simulink model "FFT_FILTER_DESIGN"  (R2020b)
settings: Solver=VariableStepAuto  StartTime=0.0  StopTime=inf  RelTol=1e-3
libraries: dspsrcs4 x2, dspxfrm3 x2, commrandsrc3 x1, simulink x1, commutil2 x1, dspmathops x1
settings Model: Creator=Qrush  LastModifiedBy=AlexKurash

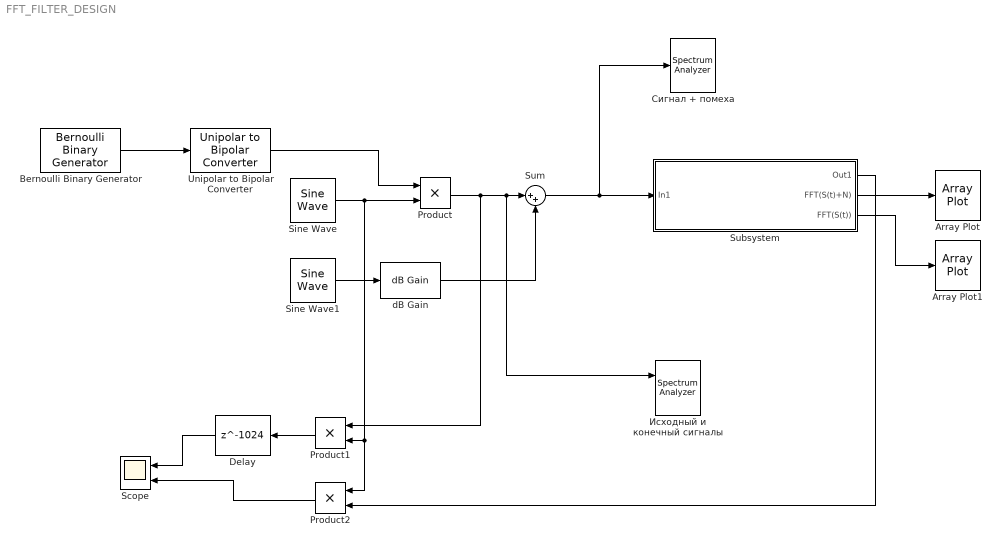
== system FFT_FILTER_DESIGN ==
  Array Plot : ArrayPlot
  Array Plot1 : ArrayPlot
  Bernoulli Binary Generator : commrandsrc3/Bernoulli Binary Generator  ProbabilityOfZero=0.5  SeedSource=Auto  Seed=0  SampleTime=1/128  SamplesPerFrame=1  OutputDataType=double  SimulateUsing=Interpreted execution
  Delay : Delay  DelayLength=1024  InitialCondition=0
  Product : Product
  Product1 : Product
  Product2 : Product
  Scope : Scope  NumInputPorts=2
  Sine Wave : dspsrcs4/Sine Wave  Amplitude=1  Frequency=200  Phase=0  SampleMode=Discrete  OutComplex=Real  CompMethod=Trigonometric fcn  TableSize=Speed  SampleTime=1/2048  SamplesPerFrame=1  ResetState=Restart at time zero  OutputFrames=off  dataType=double  wordLen=16  udDataType=sfix(16)  fracBitsMode=Best precision  numFracBits=15  OutDataTypeStr=double  LastOutDataTypeStr=double
  Sine Wave1 : dspsrcs4/Sine Wave  Amplitude=1  Frequency=224  Phase=0  SampleMode=Discrete  OutComplex=Real  CompMethod=Trigonometric fcn  TableSize=Speed  SampleTime=1/2048  SamplesPerFrame=1  ResetState=Restart at time zero  OutputFrames=off  dataType=double  wordLen=16  udDataType=sfix(16)  fracBitsMode=Best precision  numFracBits=15  OutDataTypeStr=double  LastOutDataTypeStr=double
  Subsystem : Subsystem  mask(Fourier Filtration){FFT_Length=1024, ThrValue=150}
      mask prompts: FFT_Length "FFT Length (число точек БПФ):"; ThrValue "Thresshold Value (Пороговое Значение)"
      mask help:
      | ENG: This block performs bandpass interference rejection based on the fast Fourier transform algorithm, the rejection is performed by comparing the components with the threshold level, and zeroing the components that exceed the specified threshold.
      |
      | The threshold level can be set based on graphically visualized FFT results that can be obtained from the debug ports.
      | ----------------------------------------
      | RUS: Данный блок осуществляет режекцию полосовых помех на основании алгоритма быстрого преобразования фурье, режекция осуществляется путем сравнения компонент с пороговым уровнем, и обнулением компоненты превышающих заданный порог.
      |
      | Настройку порогового уровня можно осуществить на основании графически-визуализированных результатов FFT , которые могут быть получены с портов отладки
      | ----------------------------------------
      mask Display:
      | disp ('FFT filtration')
      | port_label('input', 1, 'S(t)+N')
      | port_label('output', 1, 'S(t)')
      | port_label('output', 2, 'FFT(S(t)+N)')
      | port_label('output', 3, 'FFT(S(t))')
  Sum : Sum  Inputs=|++
  Unipolar to Bipolar Converter : commutil2/Unipolar to Bipolar Converter  M=2  polarity=Positive  dataType=Inherit via internal rule
  dB Gain : dspmathops/dB Gain  dB=-5  intype=Power
      settings: SourceProductBaseCode=DS
  Исходный и конечный сигналы : SpectrumAnalyzer  NumInputPorts=2
  Сигнал + помеха : SpectrumAnalyzer
  wires:
  Sine Wave1/1 -> dB Gain/1
  Sine Wave/1 -> Product2/1, Product1/2, Product/2
  Product/1 -> Product1/1, Исходный и конечный сигналы/1, Sum/1
  Bernoulli Binary Generator/1 -> Unipolar to Bipolar Converter/1
  Unipolar to Bipolar Converter/1 -> Product/1
  Sum/1 -> Subsystem/1(In1), Сигнал + помеха/1
  Product1/1 -> Delay/1
  Delay/1 -> Scope/1
  Product2/1 -> Scope/2
  dB Gain/1 -> Sum/2
  Subsystem/2(FFT(S(t)+N)) -> Array Plot/1
  Subsystem/3(FFT(S(t))) -> Array Plot1/1
  Subsystem/1(Out1) -> Product2/2

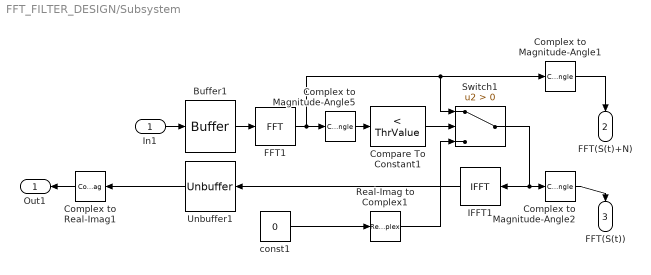
== system FFT_FILTER_DESIGN/Subsystem ==
  In1 : Inport
  Buffer1 : Buffer  N=FFT_Length  OutputFrames=off
  Compare To Constant1 : simulink/Logic and Bit Operations/Compare To Constant  relop=<  const=ThrValue  OutDataTypeStr=boolean
  Complex to Magnitude-Angle1 : ComplexToMagnitudeAngle  Output=Magnitude
  Complex to Magnitude-Angle2 : ComplexToMagnitudeAngle  Output=Magnitude
  Complex to Magnitude-Angle5 : ComplexToMagnitudeAngle  Output=Magnitude
  Complex to Real-Imag1 : ComplexToRealImag  Output=Real
  FFT1 : dspxfrm3/FFT  FFTImplementation=Auto  CompMethod=Table lookup  TableOpt=NEW  TableOptActive=Speed  BitRevOrder=off  Normalize=off  InheritFFTLength=on  FFTLength=FFT_Length  WrapInput=on  roundingMode=Floor  overflowMode=off  firstCoeffDataTypeStr=Inherit: Same word length as input  firstCoeffLastDataTypeStr=Inherit: Same word length as input  outputMin=[]  outputMax=[]
  IFFT1 : dspxfrm3/IFFT  FFTImplementation=Auto  CompMethod=Table lookup  TableOpt=NEW  TableOptActive=Speed  BitRevOrder=off  cs_in=off  Normalize=on  InheritFFTLength=on  FFTLength=FFT_Length  WrapInput=on  mode=Complex  outSamplingMode=Sample based  roundingMode=Floor  overflowMode=off  firstCoeffDataTypeStr=Inherit: Same word length as input  firstCoeffLastDataTypeStr=Inherit: Same word length as input  outputMin=[]  outputMax=[]
  Real-Imag to Complex1 : RealImagToComplex  Input=Real
  Switch1 : Switch  Criteria=u2 > Threshold
  Unbuffer1 : Unbuffer
  const1 : Constant  Value=0  OutDataTypeStr=Inherit: Inherit via back propagation
  Out1 : Outport
  FFT(S(t)+N) : Outport  Port=2
  FFT(S(t)) : Outport  Port=3
  wires:
  Buffer1/1 -> FFT1/1
  Switch1/1 -> Complex to Magnitude-Angle2/1, IFFT1/1
  In1/1 -> Buffer1/1
  IFFT1/1 -> Unbuffer1/1
  const1/1 -> Real-Imag to Complex1/1
  Complex to Magnitude-Angle5/1 -> Compare To Constant1/1
  Compare To Constant1/1 -> Switch1/2
  Unbuffer1/1 -> Complex to Real-Imag1/1
  Complex to Real-Imag1/1 -> Out1/1
  Complex to Magnitude-Angle1/1 -> FFT(S(t)+N)/1
  Complex to Magnitude-Angle2/1 -> FFT(S(t))/1
  FFT1/1 -> Switch1/1, Complex to Magnitude-Angle1/1, Complex to Magnitude-Angle5/1
  Real-Imag to Complex1/1 -> Switch1/3
